simulink model "TPGCI_STM32_2"  (R2024a)
settings: Solver=FixedStepDiscrete  StartTime=0.0  StopTime=10.0  RelTol=1e-3
undefined symbols (not defined in the file): DiscIntNeverNeededParam
libraries: slpidlib x3
settings Model: Creator=mahes  LastModifiedBy=mahes
settings OptimizationCC: DefaultParameterBehavior=Inlined  UseDivisionForNetSlopeComputation=on  GainParamInheritBuiltInType=on  UseFloatMulNetSlope=on  InlineInvariantSignals=on  PassReuseOutputArgsAs=Individual arguments  ZeroExternalMemoryAtStartup=off  ZeroInternalMemoryAtStartup=off  NoFixptDivByZeroProtection=on  EfficientFloat2IntCast=on  LifeSpan=1  OptimizeBlockOrder=speed  DifferentSizesBufferReuse=on  EfficientTunableParamExpr=on
settings DebuggingCC: ParameterTunabilityLossMsg=error
settings HardwareCC: ProdBitPerPointer=32  ProdBitPerSizeT=32  ProdBitPerPtrDiffT=32  ProdLargestAtomicInteger=Long  ProdLargestAtomicFloat=Double  ProdWordSize=32  ProdLongLongMode=on  ProdHWDeviceType=ARM Compatible->ARM Cortex-M
settings SFSimCC: MATLABDynamicMemAlloc=off
settings RTWCC: Description=Embedded Coder  SystemTargetFile=ert.tlc  TemplateMakefile=ert_default_tmf  DataTypeReplacement=CDataTypesFixedWidth
settings CodeAppCC: ForceParamTrailComments=on  IgnoreCustomStorageClasses=off  OperatorAnnotations=on  SimulinkDataObjDesc=on  SFDataObjDesc=on  CustomSymbolStrGlobalVar=rt$N$M  CustomSymbolStrType=$N$M  CustomSymbolStrFcn=$N$M$F  CustomSymbolStrMacro=$N$M  InsertBlockDesc=on
settings ERTTargetCC: TargetLangStandard=C99 (ISO)  GenerateSampleERTMain=on  IncludeMdlTerminateFcn=off  CombineSignalStateStructs=on  SupportAbsoluteTime=off  SupportComplex=off  SupportNonInlinedSFcns=on  InlinedParameterPlacement=NonHierarchical  ERTCustomFileTemplate=example_file_process.tlc  ERTFilePackagingFormat=CompactWithDataFile  MaxIdInt64=INT64_MAX  MinIdInt64=INT64_MIN  MaxIdUint64=UINT64_MAX  MaxIdInt32=INT32_MAX  MinIdInt32=INT32_MIN  MaxIdUint32=UINT32_MAX  MaxIdInt16=INT16_MAX  MinIdInt16=INT16_MIN  MaxIdUint16=UINT16_MAX  MaxIdInt8=INT8_MAX  MinIdInt8=INT8_MIN  MaxIdUint8=UINT8_MAX

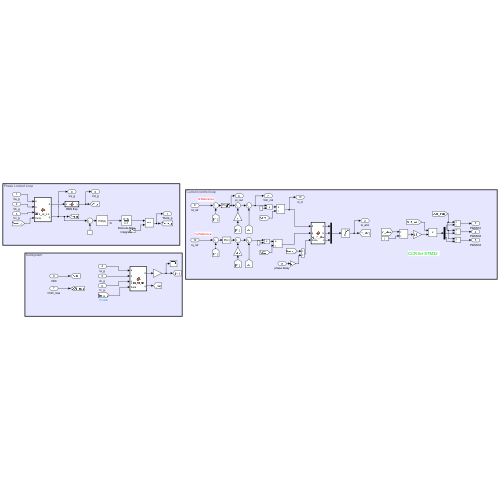
[thumbnail: Simulink's stored preview of the top-level diagram]
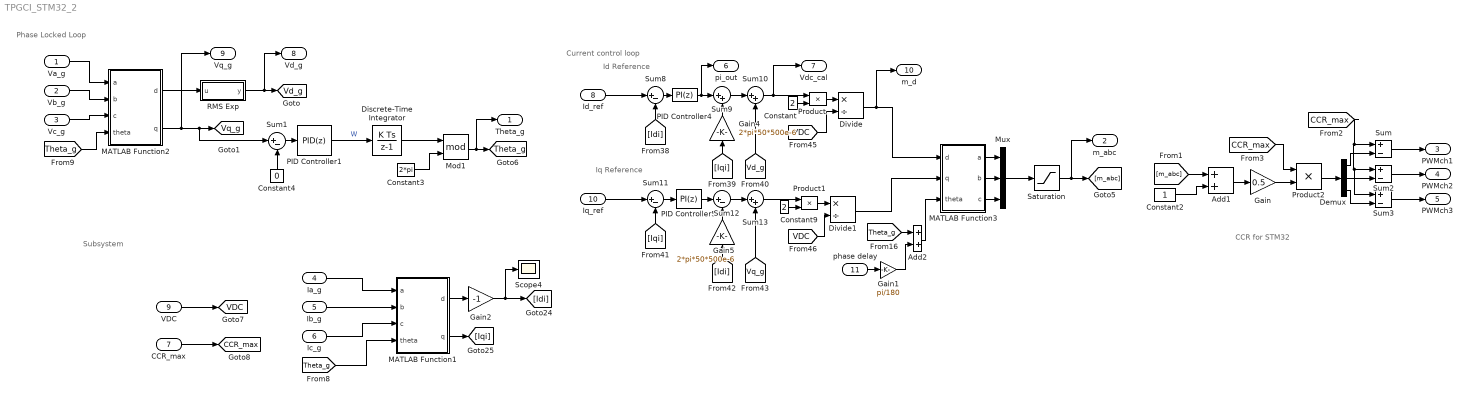
== system TPGCI_STM32_2 ==
  note: Current control loop
  note: Iq Reference
  note: Id Reference
  note: Phase Locked Loop
  note: CCR for STM32
  note: Subsystem
  Va_g : Inport
  Vb_g : Inport  Port=2
  Vc_g : Inport  Port=3
  Ia_g : Inport  Port=4
  Ib_g : Inport  Port=5
  Ic_g : Inport  Port=6
  CCR_max : Inport  Port=7
  Id_ref : Inport  Port=8
  VDC : Inport  Port=9
  Iq_ref : Inport  Port=10
  phase delay : Inport  Port=11
  Add1 : Sum
  Add2 : Sum
  Constant : Constant  Value=2
  Constant2 : Constant
  Constant3 : Constant  Value=2*pi
  Constant4 : Constant  Value=0
  Constant9 : Constant  Value=2
  Demux : Demux  Outputs=3
  Discrete-Time Integrator : DiscreteIntegrator  SampleTime=-1  ICPrevOutput=DiscIntNeverNeededParam  ICPrevScaledInput=DiscIntNeverNeededParam
  Divide : Product  Inputs=*/
  Divide1 : Product  Inputs=*/
  Gain : Gain  Gain=0.5
  Gain1 : Gain  Gain=pi/180
  Gain2 : Gain  Gain=-1
  Gain4 : Gain  Gain=2*pi*50*500e-6
  Gain5 : Gain  Gain=2*pi*50*500e-6
  MATLAB Function1 : MATLAB Function  TreatAsAtomicUnit=on
  MATLAB Function2 : MATLAB Function  TreatAsAtomicUnit=on
  MATLAB Function3 : MATLAB Function  TreatAsAtomicUnit=on
  Mod1 : Math  Operator=mod
  Mux : Mux  Inputs=3
  PID Controller1 : slpidlib/PID Controller  Controller=PID  Form=Parallel  TimeDomain=Discrete-time  UseExternalTs=off  SampleTime=4e-5  IntegratorMethod=Forward Euler  FilterMethod=Forward Euler  ControllerParametersSource=internal  P=10  I=10000  UseKiTs=off  D=0  UseExternalDerivativeSource=off  N=100  UseFilter=on  TunerSelectOption=Transfer Function Based (PID Tuner App)  InitialConditionSource=internal  InitialConditionForIntegrator=0  InitialConditionForFilter=0  DifferentiatorICPrevScaledInput=0  ExternalReset=none  TrackingMode=off  Kt=1  LimitOutput=off  SatLimitsSource=internal  UpperSaturationLimit=inf  LowerSaturationLimit=-inf  LinearizeAsGain=on  AntiWindupMode=none  Kb=1  LimitIntegrator=off  UpperIntegratorSaturationLimit=inf  LowerIntegratorSaturationLimit=-inf  POutMin=[]  POutMax=[]  IOutMin=[]  IOutMax=[]  DOutMin=[]  DOutMax=[]  NOutMin=[]  NOutMax=[]  SumOutMin=[]  SumOutMax=[]  SaturationOutMin=[]  SaturationOutMax=[]  PParamMin=[]  PParamMax=[]  IParamMin=[]  IParamMax=[]  DParamMin=[]  DParamMax=[]  NParamMin=[]  NParamMax=[]  KbParamMin=[]  KbParamMax=[]  KtParamMin=[]  KtParamMax=[]  KbOutMin=[]  KbOutMax=[]  KtOutMin=[]  KtOutMax=[]  IntegratorOutMin=[]  IntegratorOutMax=[]  FilterOutMin=[]  FilterOutMax=[]  SumI1OutMin=[]  SumI1OutMax=[]  SumI2OutMin=[]  SumI2OutMax=[]  SumI3OutMin=[]  SumI3OutMax=[]  SumI4OutMin=[]  SumI4OutMax=[]  SumDOutMin=[]  SumDOutMax=[]  DifferentiatorOutMin=[]  DifferentiatorOutMax=[]  FilterDiffOutCoefMin=[]  FilterDiffOutCoefMax=[]  ReciprocalOutMin=[]  ReciprocalOutMax=[]  SumDenOutMin=[]  SumDenOutMax=[]  SumNumOutMin=[]  SumNumOutMax=[]  DivideOutMin=[]  DivideOutMax=[]  UdiffTsProdOutMin=[]  UdiffTsProdOutMax=[]  NTsProdOutMin=[]  NTsProdOutMax=[]  UintegralTsProdOutMin=[]  UintegralTsProdOutMax=[]  UngainTsProdOutMin=[]  UngainTsProdOutMax=[]  ClampingZeroOutDataTypeStr=Inherit: Inherit via back propagation  ClampingZeroOutMin=[]  ClampingZeroOutMax=[]  FilterDenConstantOutDataTypeStr=Inherit: Inherit via back propagation  FilterDenConstantOutMin=[]  FilterDenConstantOutMax=[]  PCopyOutDataTypeStr=Inherit: Inherit via back propagation  PCopyOutMin=[]  PCopyOutMax=[]  NCopyOutDataTypeStr=Inherit: Inherit via back propagation  NCopyOutMin=[]  NCopyOutMax=[]  IntegratorContinuousStateAttributes=''  IntegratorStateMustResolveToSignalObject=off  IntegratorRTWStateStorageClass=Auto  FilterContinuousStateAttributes=''  FilterStateMustResolveToSignalObject=off  FilterRTWStateStorageClass=Auto  ParallelPVariant=InternalParameters  IdealPVariant=Disabled  IVariant=InternalParameters  DVariant=InternalParameters  IntegratorVariant=Discrete  SatVariant=Disabled  AWVariant=Passthrough  PCopyVariant=Disabled  TRVariant=Disabled  FdbkBlocksVariant=Forward  IdealPFdbkVariant=Disabled  SatFdbkVariant=Disabled  DerivativeFilterVariant=ForwardEulerFilter  NVariant=InternalParameters  NCopyVariant=Disabled  FilterICVariant=InternalICsFilter  IntegratorICVariant=InternalICs  ExternalResetVariant=Disabled  TRSumVariant=Passthrough  SumFdbkVariant=Disabled  SumVariant=Sum_PID  TsampFilterVariant=InternalTs  TsampNgainVariant=Passthrough  TsampIntegralVariant=Disabled_SignalSpec  ExternalSaturationOutDataTypeStr=Inherit: Same as second input  DerivativeSourceVariant=ErrorSignal
  PID Controller4 : slpidlib/PID Controller  Controller=PI  Form=Parallel  TimeDomain=Discrete-time  UseExternalTs=off  SampleTime=4e-5  IntegratorMethod=Forward Euler  FilterMethod=Forward Euler  ControllerParametersSource=internal  P=0.001  I=1  UseKiTs=off  D=0  UseExternalDerivativeSource=off  N=100  UseFilter=on  TunerSelectOption=Transfer Function Based (PID Tuner App)  InitialConditionSource=internal  InitialConditionForIntegrator=0  InitialConditionForFilter=0  DifferentiatorICPrevScaledInput=0  ExternalReset=none  TrackingMode=off  Kt=1  LimitOutput=on  SatLimitsSource=internal  UpperSaturationLimit=5  LowerSaturationLimit=-5  LinearizeAsGain=on  AntiWindupMode=none  Kb=1  LimitIntegrator=on  UpperIntegratorSaturationLimit=5  LowerIntegratorSaturationLimit=-5  POutMin=[]  POutMax=[]  IOutMin=[]  IOutMax=[]  DOutMin=[]  DOutMax=[]  NOutMin=[]  NOutMax=[]  SumOutMin=[]  SumOutMax=[]  SaturationOutMin=[]  SaturationOutMax=[]  PParamMin=[]  PParamMax=[]  IParamMin=[]  IParamMax=[]  DParamMin=[]  DParamMax=[]  NParamMin=[]  NParamMax=[]  KbParamMin=[]  KbParamMax=[]  KtParamMin=[]  KtParamMax=[]  KbOutMin=[]  KbOutMax=[]  KtOutMin=[]  KtOutMax=[]  IntegratorOutMin=[]  IntegratorOutMax=[]  FilterOutMin=[]  FilterOutMax=[]  SumI1OutMin=[]  SumI1OutMax=[]  SumI2OutMin=[]  SumI2OutMax=[]  SumI3OutMin=[]  SumI3OutMax=[]  SumI4OutMin=[]  SumI4OutMax=[]  SumDOutMin=[]  SumDOutMax=[]  DifferentiatorOutMin=[]  DifferentiatorOutMax=[]  FilterDiffOutCoefMin=[]  FilterDiffOutCoefMax=[]  ReciprocalOutMin=[]  ReciprocalOutMax=[]  SumDenOutMin=[]  SumDenOutMax=[]  SumNumOutMin=[]  SumNumOutMax=[]  DivideOutMin=[]  DivideOutMax=[]  UdiffTsProdOutMin=[]  UdiffTsProdOutMax=[]  NTsProdOutMin=[]  NTsProdOutMax=[]  UintegralTsProdOutMin=[]  UintegralTsProdOutMax=[]  UngainTsProdOutMin=[]  UngainTsProdOutMax=[]  ClampingZeroOutDataTypeStr=Inherit: Inherit via back propagation  ClampingZeroOutMin=[]  ClampingZeroOutMax=[]  FilterDenConstantOutDataTypeStr=Inherit: Inherit via back propagation  FilterDenConstantOutMin=[]  FilterDenConstantOutMax=[]  PCopyOutDataTypeStr=Inherit: Inherit via back propagation  PCopyOutMin=[]  PCopyOutMax=[]  NCopyOutDataTypeStr=Inherit: Inherit via back propagation  NCopyOutMin=[]  NCopyOutMax=[]  IntegratorContinuousStateAttributes=''  IntegratorStateMustResolveToSignalObject=off  IntegratorRTWStateStorageClass=Auto  FilterContinuousStateAttributes=''  FilterStateMustResolveToSignalObject=off  FilterRTWStateStorageClass=Auto  ParallelPVariant=InternalParameters  IdealPVariant=Disabled  IVariant=InternalParameters  DVariant=Disabled  IntegratorVariant=Discrete  SatVariant=Enabled  AWVariant=Passthrough  PCopyVariant=Disabled  TRVariant=Disabled  FdbkBlocksVariant=Forward  IdealPFdbkVariant=Disabled  SatFdbkVariant=Disabled  DerivativeFilterVariant=Disabled  NVariant=Disabled  NCopyVariant=Disabled_SignalSpec  FilterICVariant=Disabled  IntegratorICVariant=InternalICs  ExternalResetVariant=Disabled  TRSumVariant=Passthrough  SumFdbkVariant=Disabled  SumVariant=Sum_PI  TsampFilterVariant=InternalTs  TsampNgainVariant=Passthrough  TsampIntegralVariant=Disabled_SignalSpec  ExternalSaturationOutDataTypeStr=Inherit: Same as second input  DerivativeSourceVariant=Disabled
  PID Controller5 : slpidlib/PID Controller  Controller=PI  Form=Parallel  TimeDomain=Discrete-time  UseExternalTs=off  SampleTime=4e-5  IntegratorMethod=Forward Euler  FilterMethod=Forward Euler  ControllerParametersSource=internal  P=0.001  I=1  UseKiTs=off  D=0  UseExternalDerivativeSource=off  N=100  UseFilter=on  TunerSelectOption=Transfer Function Based (PID Tuner App)  InitialConditionSource=internal  InitialConditionForIntegrator=0  InitialConditionForFilter=0  DifferentiatorICPrevScaledInput=0  ExternalReset=none  TrackingMode=off  Kt=1  LimitOutput=off  SatLimitsSource=internal  UpperSaturationLimit=10  LowerSaturationLimit=-10  LinearizeAsGain=on  AntiWindupMode=none  Kb=1  LimitIntegrator=off  UpperIntegratorSaturationLimit=10  LowerIntegratorSaturationLimit=-10  POutMin=[]  POutMax=[]  IOutMin=[]  IOutMax=[]  DOutMin=[]  DOutMax=[]  NOutMin=[]  NOutMax=[]  SumOutMin=[]  SumOutMax=[]  SaturationOutMin=[]  SaturationOutMax=[]  PParamMin=[]  PParamMax=[]  IParamMin=[]  IParamMax=[]  DParamMin=[]  DParamMax=[]  NParamMin=[]  NParamMax=[]  KbParamMin=[]  KbParamMax=[]  KtParamMin=[]  KtParamMax=[]  KbOutMin=[]  KbOutMax=[]  KtOutMin=[]  KtOutMax=[]  IntegratorOutMin=[]  IntegratorOutMax=[]  FilterOutMin=[]  FilterOutMax=[]  SumI1OutMin=[]  SumI1OutMax=[]  SumI2OutMin=[]  SumI2OutMax=[]  SumI3OutMin=[]  SumI3OutMax=[]  SumI4OutMin=[]  SumI4OutMax=[]  SumDOutMin=[]  SumDOutMax=[]  DifferentiatorOutMin=[]  DifferentiatorOutMax=[]  FilterDiffOutCoefMin=[]  FilterDiffOutCoefMax=[]  ReciprocalOutMin=[]  ReciprocalOutMax=[]  SumDenOutMin=[]  SumDenOutMax=[]  SumNumOutMin=[]  SumNumOutMax=[]  DivideOutMin=[]  DivideOutMax=[]  UdiffTsProdOutMin=[]  UdiffTsProdOutMax=[]  NTsProdOutMin=[]  NTsProdOutMax=[]  UintegralTsProdOutMin=[]  UintegralTsProdOutMax=[]  UngainTsProdOutMin=[]  UngainTsProdOutMax=[]  ClampingZeroOutDataTypeStr=Inherit: Inherit via back propagation  ClampingZeroOutMin=[]  ClampingZeroOutMax=[]  FilterDenConstantOutDataTypeStr=Inherit: Inherit via back propagation  FilterDenConstantOutMin=[]  FilterDenConstantOutMax=[]  PCopyOutDataTypeStr=Inherit: Inherit via back propagation  PCopyOutMin=[]  PCopyOutMax=[]  NCopyOutDataTypeStr=Inherit: Inherit via back propagation  NCopyOutMin=[]  NCopyOutMax=[]  IntegratorContinuousStateAttributes=''  IntegratorStateMustResolveToSignalObject=off  IntegratorRTWStateStorageClass=Auto  FilterContinuousStateAttributes=''  FilterStateMustResolveToSignalObject=off  FilterRTWStateStorageClass=Auto  ParallelPVariant=InternalParameters  IdealPVariant=Disabled  IVariant=InternalParameters  DVariant=Disabled  IntegratorVariant=Discrete  SatVariant=Disabled  AWVariant=Passthrough  PCopyVariant=Disabled  TRVariant=Disabled  FdbkBlocksVariant=Forward  IdealPFdbkVariant=Disabled  SatFdbkVariant=Disabled  DerivativeFilterVariant=Disabled  NVariant=Disabled  NCopyVariant=Disabled_SignalSpec  FilterICVariant=Disabled  IntegratorICVariant=InternalICs  ExternalResetVariant=Disabled  TRSumVariant=Passthrough  SumFdbkVariant=Disabled  SumVariant=Sum_PI  TsampFilterVariant=InternalTs  TsampNgainVariant=Passthrough  TsampIntegralVariant=Disabled_SignalSpec  ExternalSaturationOutDataTypeStr=Inherit: Same as second input  DerivativeSourceVariant=Disabled
  Product : Product
  Product1 : Product
  Product2 : Product
  RMS Exp : MATLAB Function  TreatAsAtomicUnit=on
  Saturation : Saturate  UpperLimit=0.95  LowerLimit=-0.95
  Scope4 : Scope
  Sum : Sum  Inputs=+-
  Sum{1,8,11..12} (4 alike) : Sum  Inputs=|+-
  Sum10 : Sum  Inputs=|++
  Sum13 : Sum  Inputs=|++
  Sum2 : Sum  Inputs=+-
  Sum3 : Sum  Inputs=+-
  Sum9 : Sum  Inputs=|++
  Theta_g : Outport
  m_abc : Outport  Port=2
  PWMch1 : Outport  Port=3
  PWMch2 : Outport  Port=4
  PWMch3 : Outport  Port=5
  pi_out : Outport  Port=6
  Vdc_cal : Outport  Port=7
  Vd_g : Outport  Port=8
  Vq_g : Outport  Port=9
  m_d : Outport  Port=10
  tag scope: CCR_max=global, Theta_g=global, VDC=global, Vd_g=global, Vq_g=global
  wires:
  Sum11/1 -> PID Controller5/1
  phase delay/1 -> Gain1/1
  [VDC] -> Divide/2
  Gain1/1 -> Add2/2
  VDC/1 -> [VDC]
  MATLAB Function2/1(d) -> RMS Exp/1(u)
  [CCR_max] -> Product2/1
  Product2/1 -> Demux/1
  CCR_max/1 -> [CCR_max]
  Demux/1 -> Sum/2
  [Vd_g] -> Sum10/2
  Iq_ref/1 -> Sum11/1
  Sum9/1 -> Sum10/1
  Sum2/1 -> PWMch2/1
  [CCR_max] -> Sum/1, Sum2/1, Sum3/1
  Sum/1 -> PWMch1/1
  Divide1/1 -> MATLAB Function3/2(q)
  Constant9/1 -> Product1/2
  Sum3/1 -> PWMch3/1
  Product1/1 -> Divide1/1
  Divide/1 -> MATLAB Function3/1(d), m_d/1
  Va_g/1 -> MATLAB Function2/1(a)
  Gain4/1 -> Sum9/2
  Mod1/1 -> [Theta_g], Theta_g/1
  Demux/3 -> Sum3/2
  Constant4/1 -> Sum1/2
  [Iqi] -> Gain4/1
  Constant2/1 -> Add1/2
  Sum10/1 -> Product/1, Vdc_cal/1
  [Iqi] -> Sum11/2
  Gain5/1 -> Sum12/2
  [Theta_g] -> Add2/1
  PID Controller1/1 -> Discrete-Time Integrator/1  "W"
  [Theta_g] -> MATLAB Function2/4(theta)
  Saturation/1 -> m_abc/1, [m_abc]
  MATLAB Function2/2(q) -> Vq_g/1, [Vq_g], Sum1/1
  PID Controller5/1 -> Sum12/1
  Sum13/1 -> Product1/1
  Add1/1 -> Gain/1
  Gain/1 -> Product2/2
  Add2/1 -> MATLAB Function3/3(theta)
  [Idi] -> Sum8/2
  Product/1 -> Divide/1
  Constant/1 -> Product/2
  PID Controller4/1 -> Sum9/1, pi_out/1
  Demux/2 -> Sum2/2
  Sum12/1 -> Sum13/1
  [m_abc] -> Add1/1
  Discrete-Time Integrator/1 -> Mod1/1
  [VDC] -> Divide1/2
  Sum1/1 -> PID Controller1/1
  Vc_g/1 -> MATLAB Function2/3(c)
  RMS Exp/1(y) -> Vd_g/1, [Vd_g]
  [Vq_g] -> Sum13/2
  Vb_g/1 -> MATLAB Function2/2(b)
  Sum8/1 -> PID Controller4/1
  Constant3/1 -> Mod1/2
  Id_ref/1 -> Sum8/1
  [Idi] -> Gain5/1
  Ib_g/1 -> MATLAB Function1/2(b)
  MATLAB Function1/2(q) -> [Iqi]
  Ia_g/1 -> MATLAB Function1/1(a)
  Ic_g/1 -> MATLAB Function1/3(c)
  [Theta_g] -> MATLAB Function1/4(theta)
  MATLAB Function3/2(b) -> Mux/2
  MATLAB Function3/1(a) -> Mux/1
  MATLAB Function3/3(c) -> Mux/3
  Mux/1 -> Saturation/1
  MATLAB Function1/1(d) -> Gain2/1
  Gain2/1 -> Scope4/1, [Idi]

== matlab function TPGCI_STM32_2/MATLAB Function1 ==
  data: a input; d output; b input; c input; theta input; q output
function [d, q] = abc_to_dq(a, b, c, theta) %#codegen
% abc_to_dq - Converts abc to dq without power-invariant scaling

% Precompute constants
K = 2/3; % Non-power-invariant scaling factor
PI_2_OVER_3 = 2.094395102393195; % Precomputed 2*pi/3

% Precompute sine and cosine values
sin_theta = sin(theta);
cos_theta = cos(theta);
sin_theta_120 = sin(theta - PI_2_OVER_3);
cos_theta_120 = cos(theta - PI_2_OVER_3);
sin_theta_240 = sin(theta + PI_2_OVER_3);
cos_theta_240 = cos(theta + PI_2_OVER_3);

% Compute d and q components
d = K * (a * sin_theta + b * sin_theta_120 + c * sin_theta_240);
q = K * (a * cos_theta + b * cos_theta_120 + c * cos_theta_240);

== matlab function TPGCI_STM32_2/MATLAB Function2 ==
  data: a input; d output; b input; c input; theta input; q output
function [d, q] = abc_to_dq(a, b, c, theta) %#codegen
% abc_to_dq - Converts abc to dq without power-invariant scaling

% Precompute constants
K = 2/3; % Non-power-invariant scaling factor
PI_2_OVER_3 = 2.094395102393195; % Precomputed 2*pi/3

% Precompute sine and cosine values
sin_theta = sin(theta);
cos_theta = cos(theta);
sin_theta_120 = sin(theta - PI_2_OVER_3);
cos_theta_120 = cos(theta - PI_2_OVER_3);
sin_theta_240 = sin(theta + PI_2_OVER_3);
cos_theta_240 = cos(theta + PI_2_OVER_3);

% Compute d and q components
d = K * (a * sin_theta + b * sin_theta_120 + c * sin_theta_240);
q = K * (a * cos_theta + b * cos_theta_120 + c * cos_theta_240);

== matlab function TPGCI_STM32_2/MATLAB Function3 ==
  data: d input; a output; q input; theta input; b output; c output
function [a, b, c] = dq_to_abc(d, q, theta) %#codegen
% dq_to_abc - Converts dq to abc without power-invariant scaling

% Precompute constants
PI_2_OVER_3 = 2.094395102393195; % Precomputed 2*pi/3

% Precompute sine and cosine values
sin_theta = sin(theta);
cos_theta = cos(theta);
sin_theta_120 = sin(theta - PI_2_OVER_3);
cos_theta_120 = cos(theta - PI_2_OVER_3);
sin_theta_240 = sin(theta + PI_2_OVER_3);
cos_theta_240 = cos(theta + PI_2_OVER_3);

% Compute a, b, c phase values
a = (d * sin_theta + q * cos_theta);
b = (d * sin_theta_120 + q * cos_theta_120);
c = (d * sin_theta_240 + q * cos_theta_240);

== matlab function TPGCI_STM32_2/RMS Exp ==
  settings: updateMethod=DISCRETE
  data: y output; u input
function y = movingRMSExp(u)
    % y = movingRMSExp(u, alpha)
    % This function computes the exponential moving RMS of the input signal `u`.
    % The parameter `alpha` is the smoothing factor (0 < alpha <= 1).
    % A higher `alpha` gives more weight to recent values.

    % Persistent variables to maintain state between calls
    persistent rmsSquared

    % Initialize the exponential moving RMS on the first call
    if isempty(rmsSquared)
        rmsSquared = u^2; % Initialize with the square of the first value
    end

    % Update the exponentially weighted RMS squared
    rmsSquared = 0.01 * u^2 + (1 - 0.01) * rmsSquared;

    % Compute the RMS as the square root of the weighted sum
    y = sqrt(rmsSquared);
end
